simulink model "sm_stewart_platform"  (R2021b)
settings: Solver=ode45  StartTime=0.0  StopTime=40  MaxStep=0.2  RelTol=1e-3  EnableMultiTasking=on
model workspace (MAT data in the model file):
  g_density = 5
values from neighbouring files (symbols this model uses):
  B = zeros(3, 6)    [sm_stewart_platform_setup.m]
  nom_length = params.lower_leg_length + params.upper_leg_length +      2 * params.flange_length    [sm_stewart_platform_setup.m]
  P = rotation3(-pi/3, [0 0 1]) * P    [sm_stewart_platform_setup.m]
  s = cos(angle / 2)    [sm_stewart_platform_setup.m]
undefined symbols (not defined in the file or in its folder): X, Y, Z
libraries: sm_lib x20, sm_stewart_platform_lib x8, nesl_utility x4
(part 2 of 3)

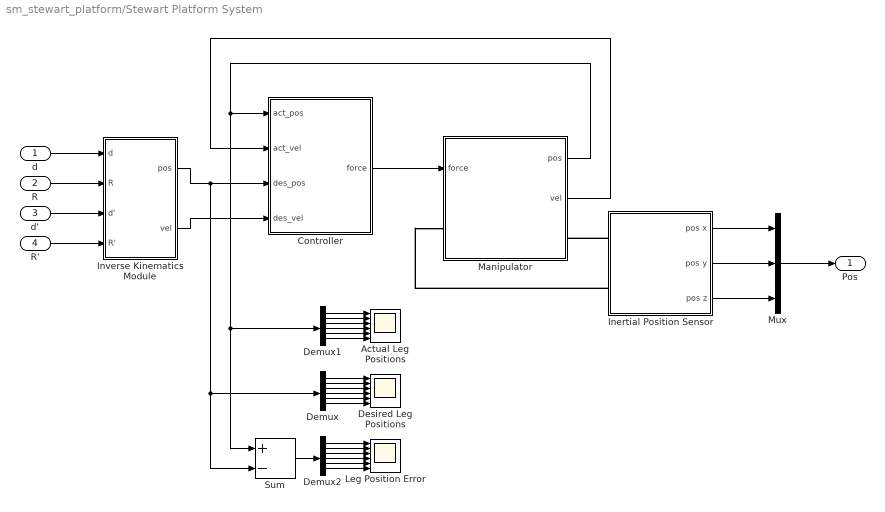
== system sm_stewart_platform/Stewart Platform System ==
  d : Inport
  R : Inport  Port=2
  d' : Inport  Port=3
  R' : Inport  Port=4
  Actual Leg Positions : Scope  NumInputPorts=6
  Controller : Subsystem  mask(PID Controller){Kp=Kp, Ki=Ki, Kd=Kd}
      mask prompts: Kp "Proportional Gain"; Ki "Integral Gain"; Kd "Derivative Gain"
      mask help:
      | Generates an actuation output based on a desired trajectory and an actual trajectory, using a generic proportional-integral-derivative (PID) control law.  The three control gains are specified through parameters.
      |
      | Both the desired and actual trajectories are specified by separate position and velocity input signals.  The controller is generic and can control to trajectories through state spaces of arbitrary dimension; the only requirement is that all four inputs have the same dimension.
      mask Help:
      | A <em>PID Controller</em> generates an actuation output based on a desired trajectory and an actual trajectory, using a generic proportional-integral-derivative (PID) control law.  The three control gains are specified through parameters.
      | 
      | Both the desired and actual trajectories are specified by separate position and velocity input signals.  The controller is generic and can control to trajectories through state spaces of arbitrary dimension; the only requirement is that all four inputs have the same dimension.
      | 
      | This block is not specific to the Stewart platform and could serve in any general purpose control library.  For the Stewart platform application, the trajectories are all through the 6-D leg-position space.
      | 
      | <h3>Gains</h3>
      | 
      | The parameters specify the gains of the controller.
      | 
      | <ul>
      | 
      | <li> <b>Proportional Gain</b> The gain that determines the strength of the control actuation in response to current deviations between actual and desired positions.  This affects the responsiveness of the controller but can lead to instability if set too high.
      | 
      | <li> <b>Integral Gain</b> The gain that determines the strength of the control actuation in response to deviations between actual and desired positions that persist over time.  A nonzero integral term is often necessary to avoid <em>droop</em> (steady-state error).  Higher values reduce the transient response of the controller but can cause overshoot in the controlled position.
      | 
      | <li> <b>Derivative Gain</b> The gain that determines the strength of the control actuation in response to the derivative of the deviations between actual and desired positions.  This is a damping component used to reduce overshoot in the controlled position; the tradeoff is that it reduces the transient response of the controller.  Higher values increase the stiffness of the system and can lead to instability.
      | 
      | </ul>
      | 
      | 
      | <h3>Ports</h3>
      | 
      | <ul>
      | 
      | <li> <b>act_pos</b> The current actual position of the plant.
      | 
      | <li> <b>act_pos</b> The current actual velocity of the plant.  This should be the time derivative of the <em>act_pos</em> signal.
      | 
      | <li> <b>des_pos</b> The current desired position of the plant.
      | 
      | <li> <b>des_pos</b> The current desired velocity of the plant.  This should be the time derivative of the <em>des_pos</em> signal.
      | 
      | </ul>
  Demux : Demux  Outputs=6
  Demux1 : Demux  Outputs=6
  Demux2 : Demux  Outputs=6
  Desired Leg Positions : Scope  NumInputPorts=6
  Inertial Position Sensor : Subsystem
  Inverse Kinematics Module : Subsystem  mask(Stewart Platform Inverse Kinematics){}
      mask help:
      | Performs the essential inverse kinematic computations for a Stewart platform manipulator.
      |
      | Given a desired dynamic state of a Stewart platform manipulator specified by a 3-D rigid transformation from the gripper frame to the base reference frame, and the first time derivative of this transformation, this block computes the positions and velocities of the prismatic primitives of the six cylindrical leg joints necessary to achieve the desired dynamic state.
      mask Help:
      | A <em>Stewart Platform Inverse Kinematics</em> performs the essential inverse kinematic computations for a Stewart platform manipulator.
      | 
      | Given a desired dynamic state of a Stewart platform manipulator specified by a 3-D rigid transformation from the gripper frame to the base reference frame, and the first time derivative of this transformation, this block computes the positions and velocities of the prismatic primitives of the six cylindrical leg joints necessary to achieve the desired dynamic state.
      | 
      | <h3>Manipulator Transformation</h3>
      | 
      | The desired dynamic state of a Stewart platform manipulator may be specified by a single 3-D rigid transformation, called the <em>manipulator transformation</em>, and its time derivative.  The transformation is from <em>gripper</em> frame to <em>base</em> frame coordinates.  The base frame is attached to the base plate of the manipulator.  Its origin is located at the center of the base, and the z-axis points directly upward.  The gripper frame is located somewhere directly above the center of platform plate of the manipulator, and is aligned with the base frame when the positions of the prismatic primitives of all six cylindrical leg joints are equal.
      | 
      | In the following discussions, let <b>R</b> and <b>d</b> specify the rotation matrix and displacement vector, respectively, of the manipulator transformation. That is, <b>d</b> is the origin of the gripper frame specified in base frame coordinates, and the columns of <b>R</b> are the canonical <b>i</b>, <b>j</b>, and <b>k</b> vectors of the gripper frame resolved in base frame coordinates.
      | Let <b>R'</b> and <b>d'</b> be the first time derivatives of <b>R</b> and <b>d</b>, respectively.
      | 
      | <h3>Inverse Kinematics</h3>
      | 
      | Each of the six legs of the manipulator is attached between a pair of universal joints: one on the base plate and one on the platform plate.  Each leg has an internal knee joint with a sensed and actuated prismatic primitive.
      | Let <em>q_i</em> and <em>q_i'</em> be the position and velocity of this primitive on Leg <em>i</em>.  Let <em>L0</em> denote the <em>nominal</em> lengths of the legs.  This is the length of a leg when its prismatic primitive is at the zero position.
      | 
      | The goal of the inverse kinematics computation is to determine the values of <em>q_i</em> and <em>q_i'</em> for i = 1, ..., 6 needed to achieve a particular manipulator transformation and its derivative.
      | 
      | The key to understanding the inverse kinematics computations is to consider the positions of the centers of the pairs of universal joints.  (These points are the centers of the crosspieces visible in the visualization of the manipulator.)
      | 
      | Let <b>b</b>_i and <b>p</b>_i be the 3-D points specifying the center of the universal joints on the base and platform plates, respectively, to which Leg <em>i</em> is connected. <b>b</b>_i is specified in base frame coordinates, and <b>p</b>_i is specified in gripper frame coordinates.  Then the desired position of the prismatic primitive of the knee joint of Leg <em>i</em> is given by
      | 
      | <em>q_i</em> = || <b>R</b> <b>p</b>_i + <b>d</b> - <b>b</b>_i || - <em>L0</em>.
      | 
      | Denote the vector within the norm expression above as <b>o</b>_i (<b>o</b> for <em>offset</em>).
      | 
      | The desired velocity of the prismatic primitive of the knee joint of Leg <em>i</em> is obtained by differentiating the expression for <em>q_i</em>. Noting that <b>p</b>_i, <b>b</b>_i, and <em>L0</em> are constant, the result is:
      | 
      | <em>q_i'</em> = [ (<b>R'</b> <b>p</b>_i + <b>d'</b>) . <b>o</b>_i ] / || <b>o</b>_i ||.
      | 
      | Note that the denominator of this expression is equal to the vector norm in the expression for <em>q_i</em>.
      | 
      | This block computes the values of all six prismatic primitive positions and velocities according to the expressions above.  The computation of the (constant) <b>p</b>_i and <b>b</b>_i points is highly dependent on the manipulator kinematics and done in the mask initialization of the containing <em>Stewart Platform System</em> block.
      | 
      | <h3>Ports</h3>
      | 
      | <ul>
      | 
      | <li> <b>d</b> The displacement vector of the desired manipulator transformation (see above) in units of centimeters.
      | 
      | <li> <b>R</b> The rotation matrix of the desired manipulator transformation (see above).
      | 
      | <li> <b>d'</b> The time derivative of the displacement vector of the desired manipulator transformation in units of centimeters/second.
      | 
      | <li> <b>R'</b> The time derivative of the rotation matrix of the desired manipulator transformation.
      | 
      | <li> <b>pos</b> The computed positions of the prismatic primitives of the six leg joints, as a 6 x 1 vector in units of centimeters.
      | 
      | <li> <b>vel</b> The computed velocities of the prismatic primitives of the six leg joints, as a 6 x 1 vector in units of centimeters/second.
      | 
      | 
      | </ul>
      | 
      | <!--  LocalWords:  ith pos vel
      |  -->
  Leg Position Error : Scope  NumInputPorts=6
  Manipulator : Subsystem  mask(Stewart Platform Manipulator){}
      mask help: Models the mechanical portion of a complete Stewart platform manipulator system: the manipulator itself. Almost all of the Simscape Multibody blocks of the full system are contained in the manipulator subsystem.
      mask Help:
      | A <em>Stewart Platform Manipulator</em> models the mechanical portion of a complete Stewart platform manipulator system: the manipulator itself.  Almost all of the Simscape Multibody blocks of the full system are contained in the manipulator subsystem.
      | 
      | The manipulator subsystem exposes two frames: the world frame, to which the base is anchored, and the gripper frame, which is the frame at the distil end of the end effector.  Typically, a user wants to control the manipulator transformation, which is the 3-D rigid transformation from the gripper frame to the world frame.
      | 
      | The manipulator subsystem has no internal control.  However, it reports the positions and velocities of the prismatic primitives of all six cylindrical leg joints as output signals and takes the actuation forces to be applied to these primitives as input signals.  When connected to an appropriate controller, these signals are sufficient to provide any of a variety of control schemes for the manipulator.
      | 
      | <h3>Parameterization</h3>
      | 
      | The manipulator is highly parameterized.  Most of the physical dimensions of its component pieces can be controlled via parameters.  These parameters are all defined in the containing <em>Stewart Platform System</em>.  The manipulator's parameters are inherited from that block; they are not defined explicitly in this block's mask.  The parameters are also needed for the <em>Stewart Platform Inverse Kinematics</em> block.
      | 
      | See the documentation of the <em>Stewart Platform System</em> block for details.
      | 
      | <h3>Ports</h3>
      | 
      | <ul>
      | 
      | <li> <b>gripper</b> The gripper frame.  This frame is fixed at the distil end of the end effector attached to the platform plate of the Stewart platform manipulator.  It is identified with a frame glyph in the visualization of the manipulator.  Typically, a user of the manipulator wants to control the pose of this frame, with respect to a reference frame such as world.
      | 
      | <li> <b>world</b> The world frame.  This is also the reference frame of the base plate of the Stewart platform manipulator, which is rigidly attached to the world frame.
      | 
      | <li><b>pos</b> The positions of the prismatic primitives of the six leg joints as a 6 x 1 output signal in units of centimeters.
      | 
      | <li><b>vel</b> The velocities of the prismatic primitives of the six leg joints as a 6 x 1 output signal in units of centimeters/second.
      | 
      | <li><b>force</b> The actuation forces applied to the prismatic primitives of the six leg joints as a 6 x 1 input signal in units of Newtons.
      | 
      | </ul>
      | 
      | <!--  LocalWords:  Eff IC Ctrl pos vel
      |  -->
      mask Display:
      | image('sm_stewart_platform_manipulator.png')
      | color('white')
      | port_label('LConn', 1, 'world')
      | port_label('RConn', 1, 'gripper')
      | color('yellow')
      | port_label('Input', 1, 'force')
      | port_label('Output', 1, 'pos')
      | port_label('Output', 2, 'vel')
  Mux : Mux  Inputs=3
  Sum : Sum  Inputs=+-
  Pos : Outport  VectorParamsAs1DForOutWhenUnconnected=off
  wires:
  Manipulator/2(vel) -> Controller/2(act_vel)
  d/1 -> Inverse Kinematics Module/1(d)
  R/1 -> Inverse Kinematics Module/2(R)
  Demux/1 -> Desired Leg Positions/1
  Demux/2 -> Desired Leg Positions/2
  Demux/3 -> Desired Leg Positions/3
  Demux/4 -> Desired Leg Positions/4
  Demux/5 -> Desired Leg Positions/5
  Demux/6 -> Desired Leg Positions/6
  Demux1/1 -> Actual Leg Positions/1
  Demux1/2 -> Actual Leg Positions/2
  Demux1/3 -> Actual Leg Positions/3
  Demux1/4 -> Actual Leg Positions/4
  Demux1/5 -> Actual Leg Positions/5
  Demux1/6 -> Actual Leg Positions/6
  Demux2/1 -> Leg Position Error/1
  Demux2/2 -> Leg Position Error/2
  Demux2/3 -> Leg Position Error/3
  Demux2/4 -> Leg Position Error/4
  Demux2/5 -> Leg Position Error/5
  Demux2/6 -> Leg Position Error/6
  Sum/1 -> Demux2/1
  d'/1 -> Inverse Kinematics Module/3(d')
  R'/1 -> Inverse Kinematics Module/4(R')
  Controller/1(force) -> Manipulator/1(force)
  Manipulator/1(pos) -> Controller/1(act_pos), Demux1/1, Sum/1
  Inertial Position Sensor/1(pos x) -> Mux/1
  Inertial Position Sensor/2(pos y) -> Mux/2
  Inertial Position Sensor/3(pos z) -> Mux/3
  Mux/1 -> Pos/1
  Inverse Kinematics Module/2(vel) -> Controller/4(des_vel)
  Inverse Kinematics Module/1(pos) -> Controller/3(des_pos), Sum/2, Demux/1
  connections:
  Inertial Position Sensor/LConn1 -- Manipulator/RConn1
  Inertial Position Sensor/LConn2 -- Manipulator/LConn1

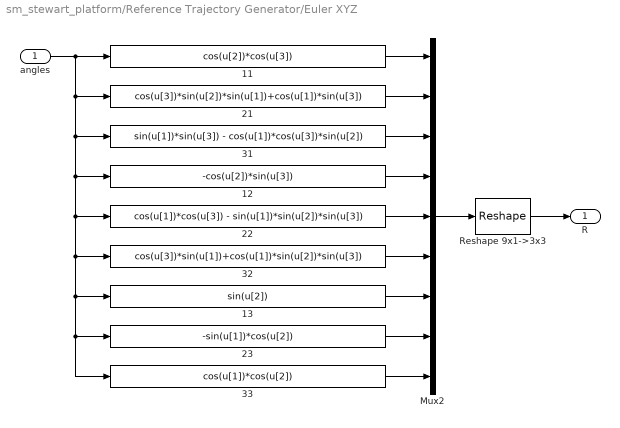
== system sm_stewart_platform/Reference Trajectory Generator/Euler XYZ ==
  angles : Inport
  11 : Fcn  Expr=cos(u[2])*cos(u[3])
  12 : Fcn  Expr=-cos(u[2])*sin(u[3])
  13 : Fcn  Expr=sin(u[2])
  21 : Fcn  Expr=cos(u[3])*sin(u[2])*sin(u[1])+cos(u[1])*sin(u[3])
  22 : Fcn  Expr=cos(u[1])*cos(u[3]) - sin(u[1])*sin(u[2])*sin(u[3])
  23 : Fcn  Expr=-sin(u[1])*cos(u[2])
  31 : Fcn  Expr=sin(u[1])*sin(u[3]) - cos(u[1])*cos(u[3])*sin(u[2])
  32 : Fcn  Expr=cos(u[3])*sin(u[1])+cos(u[1])*sin(u[2])*sin(u[3])
  33 : Fcn  Expr=cos(u[1])*cos(u[2])
  Mux2 : Mux  Inputs=9
  Reshape 9x1->3x3 : Reshape  OutputDimensionality=Customize  OutputDimensions=[3,3]
  R : Outport  VectorParamsAs1DForOutWhenUnconnected=off
  wires:
  angles/1 -> 23/1, 33/1, 13/1, 32/1, 22/1, 12/1, 31/1, 21/1, 11/1
  33/1 -> Mux2/9
  23/1 -> Mux2/8
  13/1 -> Mux2/7
  32/1 -> Mux2/6
  22/1 -> Mux2/5
  12/1 -> Mux2/4
  31/1 -> Mux2/3
  21/1 -> Mux2/2
  11/1 -> Mux2/1
  Mux2/1 -> Reshape 9x1->3x3/1
  Reshape 9x1->3x3/1 -> R/1

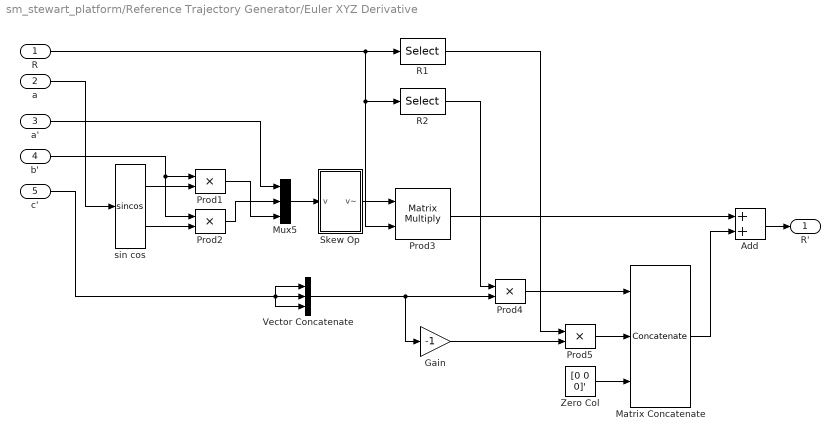
== system sm_stewart_platform/Reference Trajectory Generator/Euler XYZ Derivative ==
  R : Inport
  a : Inport  Port=2
  a' : Inport  Port=3
  b' : Inport  Port=4
  c' : Inport  Port=5
  Add : Sum
  Gain : Gain  Gain=-1
  Matrix Concatenate : Concatenate  NumInputs=3  Mode=Multidimensional array  ConcatenateDimension=2
  Mux5 : Mux  Inputs=3
  Prod{1..2,4..5} (4 alike) : Product  RndMeth=Zero
  Prod3 : Product  Multiplication=Matrix(*)  RndMeth=Zero
  R1 : Selector  NumberOfDimensions=2  InputPortWidth=3  IndexOptions=Select all,Index vector (dialog)  Indices=[1 3],1  OutputSizes=1,1
  R2 : Selector  NumberOfDimensions=2  InputPortWidth=3  IndexOptions=Select all,Index vector (dialog)  Indices=[1 3],2  OutputSizes=1,1
  Skew Op : Subsystem
  Vector Concatenate : Concatenate  NumInputs=3  Mode=Multidimensional array
  Zero Col : Constant  Value=[0 0 0]'
  sin cos : Trigonometry  Operator=sincos
  R' : Outport  VectorParamsAs1DForOutWhenUnconnected=off
  wires:
  a/1 -> sin cos/1
  sin cos/1 -> Prod1/2
  sin cos/2 -> Prod2/2
  b'/1 -> Prod2/1, Prod1/1
  a'/1 -> Mux5/1
  Prod2/1 -> Mux5/2
  Prod1/1 -> Mux5/3
  Mux5/1 -> Skew Op/1(v)
  Vector Concatenate/1 -> Prod4/2, Gain/1
  R2/1 -> Prod4/1
  Gain/1 -> Prod5/2
  Zero Col/1 -> Matrix Concatenate/3
  Prod5/1 -> Matrix Concatenate/2
  Prod4/1 -> Matrix Concatenate/1
  R1/1 -> Prod5/1
  Prod3/1 -> Add/1
  Matrix Concatenate/1 -> Add/2
  Add/1 -> R'/1
  R/1 -> R1/1, Prod3/2, R2/1
  Skew Op/1(v~) -> Prod3/1
  c'/1 -> Vector Concatenate/2, Vector Concatenate/1, Vector Concatenate/3

== system sm_stewart_platform/Reference Trajectory Generator/Rx sinusoid ==
  t : Inport
  Add : Sum  Inputs=|++
  Add2 : Sum  Inputs=++|
  amp1 : Gain  Gain=A
  amp2 : Gain  Gain=w*A*pi/180
  deg2rad : Gain  Gain=pi/180
  freq : Gain  Gain=w
  offset : Constant  Value=k  VectorParams1D=off
  phase : Constant  Value=p  VectorParams1D=off
  sin cos : Trigonometry  Operator=sincos
  f : Outport  VectorParamsAs1DForOutWhenUnconnected=off
  f' : Outport  Port=2  VectorParamsAs1DForOutWhenUnconnected=off
  wires:
  t/1 -> freq/1
  Add/1 -> deg2rad/1
  phase/1 -> Add/2
  amp2/1 -> f'/1
  Add2/1 -> f/1
  offset/1 -> Add2/1
  sin cos/1 -> amp1/1
  sin cos/2 -> amp2/1
  amp1/1 -> Add2/2
  freq/1 -> Add/1
  deg2rad/1 -> sin cos/1

== system sm_stewart_platform/Reference Trajectory Generator/Ry sinusoid ==
  t : Inport
  Add : Sum  Inputs=|++
  Add2 : Sum  Inputs=++|
  amp1 : Gain  Gain=A
  amp2 : Gain  Gain=w*A*pi/180
  deg2rad : Gain  Gain=pi/180
  freq : Gain  Gain=w
  offset : Constant  Value=k  VectorParams1D=off
  phase : Constant  Value=p  VectorParams1D=off
  sin cos : Trigonometry  Operator=sincos
  f : Outport  VectorParamsAs1DForOutWhenUnconnected=off
  f' : Outport  Port=2  VectorParamsAs1DForOutWhenUnconnected=off
  wires:
  t/1 -> freq/1
  Add/1 -> deg2rad/1
  phase/1 -> Add/2
  amp2/1 -> f'/1
  Add2/1 -> f/1
  offset/1 -> Add2/1
  sin cos/1 -> amp1/1
  sin cos/2 -> amp2/1
  amp1/1 -> Add2/2
  freq/1 -> Add/1
  deg2rad/1 -> sin cos/1

== system sm_stewart_platform/Reference Trajectory Generator/Rz sinusoid ==
  t : Inport
  Add : Sum  Inputs=|++
  Add2 : Sum  Inputs=++|
  amp1 : Gain  Gain=A
  amp2 : Gain  Gain=w*A*pi/180
  deg2rad : Gain  Gain=pi/180
  freq : Gain  Gain=w
  offset : Constant  Value=k  VectorParams1D=off
  phase : Constant  Value=p  VectorParams1D=off
  sin cos : Trigonometry  Operator=sincos
  f : Outport  VectorParamsAs1DForOutWhenUnconnected=off
  f' : Outport  Port=2  VectorParamsAs1DForOutWhenUnconnected=off
  wires:
  t/1 -> freq/1
  Add/1 -> deg2rad/1
  phase/1 -> Add/2
  amp2/1 -> f'/1
  Add2/1 -> f/1
  offset/1 -> Add2/1
  sin cos/1 -> amp1/1
  sin cos/2 -> amp2/1
  amp1/1 -> Add2/2
  freq/1 -> Add/1
  deg2rad/1 -> sin cos/1

== system sm_stewart_platform/Reference Trajectory Generator/dx sinusoid ==
  t : Inport
  Add : Sum  Inputs=|++
  Add2 : Sum  Inputs=++|
  amp1 : Gain  Gain=A
  amp2 : Gain  Gain=w*A*pi/180
  deg2rad : Gain  Gain=pi/180
  freq : Gain  Gain=w
  offset : Constant  Value=k  VectorParams1D=off
  phase : Constant  Value=p  VectorParams1D=off
  sin cos : Trigonometry  Operator=sincos
  f : Outport  VectorParamsAs1DForOutWhenUnconnected=off
  f' : Outport  Port=2  VectorParamsAs1DForOutWhenUnconnected=off
  wires:
  t/1 -> freq/1
  Add/1 -> deg2rad/1
  phase/1 -> Add/2
  amp2/1 -> f'/1
  Add2/1 -> f/1
  offset/1 -> Add2/1
  sin cos/1 -> amp1/1
  sin cos/2 -> amp2/1
  amp1/1 -> Add2/2
  freq/1 -> Add/1
  deg2rad/1 -> sin cos/1

== system sm_stewart_platform/Reference Trajectory Generator/dy sinusoid ==
  t : Inport
  Add : Sum  Inputs=|++
  Add2 : Sum  Inputs=++|
  amp1 : Gain  Gain=A
  amp2 : Gain  Gain=w*A*pi/180
  deg2rad : Gain  Gain=pi/180
  freq : Gain  Gain=w
  offset : Constant  Value=k  VectorParams1D=off
  phase : Constant  Value=p  VectorParams1D=off
  sin cos : Trigonometry  Operator=sincos
  f : Outport  VectorParamsAs1DForOutWhenUnconnected=off
  f' : Outport  Port=2  VectorParamsAs1DForOutWhenUnconnected=off
  wires:
  t/1 -> freq/1
  Add/1 -> deg2rad/1
  phase/1 -> Add/2
  amp2/1 -> f'/1
  Add2/1 -> f/1
  offset/1 -> Add2/1
  sin cos/1 -> amp1/1
  sin cos/2 -> amp2/1
  amp1/1 -> Add2/2
  freq/1 -> Add/1
  deg2rad/1 -> sin cos/1

== system sm_stewart_platform/Reference Trajectory Generator/dz sinusoid ==
  t : Inport
  Add : Sum  Inputs=|++
  Add2 : Sum  Inputs=++|
  amp1 : Gain  Gain=A
  amp2 : Gain  Gain=w*A*pi/180
  deg2rad : Gain  Gain=pi/180
  freq : Gain  Gain=w
  offset : Constant  Value=k  VectorParams1D=off
  phase : Constant  Value=p  VectorParams1D=off
  sin cos : Trigonometry  Operator=sincos
  f : Outport  VectorParamsAs1DForOutWhenUnconnected=off
  f' : Outport  Port=2  VectorParamsAs1DForOutWhenUnconnected=off
  wires:
  t/1 -> freq/1
  Add/1 -> deg2rad/1
  phase/1 -> Add/2
  amp2/1 -> f'/1
  Add2/1 -> f/1
  offset/1 -> Add2/1
  sin cos/1 -> amp1/1
  sin cos/2 -> amp2/1
  amp1/1 -> Add2/2
  freq/1 -> Add/1
  deg2rad/1 -> sin cos/1

== system sm_stewart_platform/Stewart Platform System/Controller ==
  act_pos : Inport
  act_vel : Inport  Port=2
  des_pos : Inport  Port=3
  des_vel : Inport  Port=4
  D : Gain  Gain=Kd  SaturateOnIntegerOverflow=on  OutDataTypeStr=Inherit: Same as input  ParamDataTypeStr=Inherit: Same as input
  I : Gain  Gain=Ki  SaturateOnIntegerOverflow=on  OutDataTypeStr=Inherit: Same as input  ParamDataTypeStr=Inherit: Same as input
  Integrator : Integrator  ZeroCross=off
  P : Gain  Gain=Kp  SaturateOnIntegerOverflow=on  OutDataTypeStr=Inherit: Same as input  ParamDataTypeStr=Inherit: Same as input
  Sum : Sum  Inputs=-+|  InputSameDT=on  SaturateOnIntegerOverflow=on  OutDataTypeStr=Inherit: Same as first input
  Sum1 : Sum  Inputs=+++  InputSameDT=on  SaturateOnIntegerOverflow=on  OutDataTypeStr=Inherit: Same as first input
  Sum2 : Sum  Inputs=-+|  InputSameDT=on  SaturateOnIntegerOverflow=on  OutDataTypeStr=Inherit: Same as first input
  force : Outport  VectorParamsAs1DForOutWhenUnconnected=off
  wires:
  Sum2/1 -> D/1
  D/1 -> Sum1/3
  Integrator/1 -> I/1
  P/1 -> Sum1/1
  I/1 -> Sum1/2
  Sum/1 -> P/1, Integrator/1
  act_pos/1 -> Sum/1
  des_pos/1 -> Sum/2
  Sum1/1 -> force/1
  act_vel/1 -> Sum2/1
  des_vel/1 -> Sum2/2

== system sm_stewart_platform/Stewart Platform System/Inertial Position Sensor ==
  note: `
  Pos X Converter : nesl_utility/PS-Simulink Converter  PhysicalDomain=network_engine_domain  SubClassName=ps_output  LeftPortType=input  RightPortType=output  PseudoPeriodic=off  Frequencies=[]  Unit=cm  AffineConversion=off
      settings: SourceProductBaseCode=PW,SS
  Pos Y Converter1 : nesl_utility/PS-Simulink Converter  PhysicalDomain=network_engine_domain  SubClassName=ps_output  LeftPortType=input  RightPortType=output  PseudoPeriodic=off  Frequencies=[]  Unit=cm  AffineConversion=off
      settings: SourceProductBaseCode=PW,SS
  Pos Z Converter2 : nesl_utility/PS-Simulink Converter  PhysicalDomain=network_engine_domain  SubClassName=ps_output  LeftPortType=input  RightPortType=output  PseudoPeriodic=off  Frequencies=[]  Unit=cm  AffineConversion=off
      settings: SourceProductBaseCode=PW,SS
  Transform Sensor : sm_lib/Frames and Transforms/Transform Sensor  MeasurementFrame=World  SenseAngle=off  SenseAxis=off  SenseAngle1=off  SenseAngle2=off  SenseAngle3=off  SenseQ=off  SenseR=off  SenseOmegaX=off  SenseOmegaY=off  SenseOmegaZ=off  SenseOmega1=off  SenseOmega2=off  SenseOmega3=off  SenseQDot=off  SenseRDot=off  SenseAlphaX=off  SenseAlphaY=off  SenseAlphaZ=off  SenseAlpha1=off  SenseAlpha2=off  SenseAlpha3=off  SenseQDDot=off  SenseRDDot=off  SenseX=on  SenseY=on  SenseZ=on  SenseRad=off  SenseAzim=off  SenseDist=off  SenseInc=off  SenseXDot=off  SenseYDot=off  SenseZDot=off  SenseRadDot=off  SenseAzimDot=off  SenseDistDot=off  SenseIncDot=off  SenseXDDot=off  SenseYDDot=off  SenseZDDot=off  SenseRadDDot=off  SenseAzimDDot=off  SenseDistDDot=off  SenseIncDDot=off
  gripper : PMIOPort  Side=Left
  world : PMIOPort  Port=2  Side=Left
  pos x : Outport  VectorParamsAs1DForOutWhenUnconnected=off
  pos y : Outport  Port=2  VectorParamsAs1DForOutWhenUnconnected=off
  pos z : Outport  Port=3  VectorParamsAs1DForOutWhenUnconnected=off
  wires:
  Pos Z Converter2/1 -> pos z/1
  Pos Y Converter1/1 -> pos y/1
  Pos X Converter/1 -> pos x/1
  connections:
  world/RConn1 -- Transform Sensor/LConn1
  gripper/RConn1 -- Transform Sensor/RConn1
  Pos Z Converter2/LConn1 -- Transform Sensor/RConn4
  Pos Y Converter1/LConn1 -- Transform Sensor/RConn3
  Transform Sensor/RConn2 -- Pos X Converter/LConn1

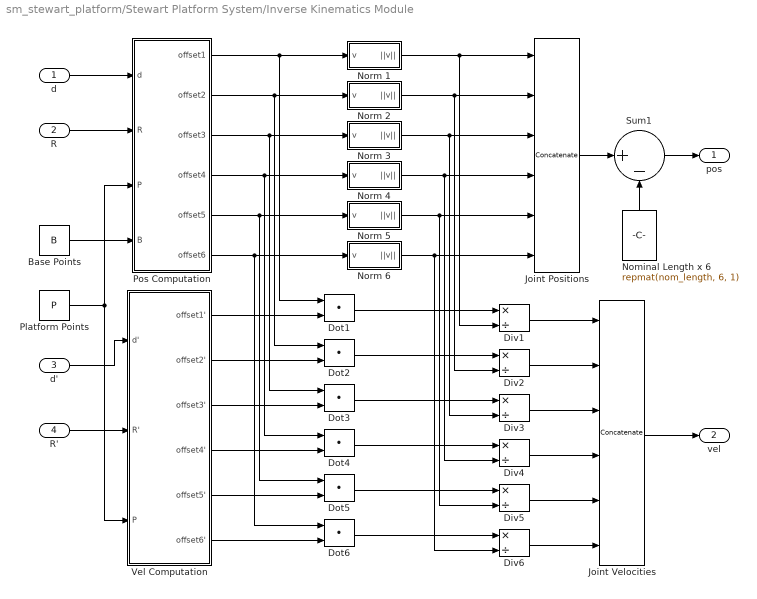
== system sm_stewart_platform/Stewart Platform System/Inverse Kinematics Module ==
  d : Inport
  R : Inport  Port=2
  d' : Inport  Port=3
  R' : Inport  Port=4
  Base Points : Constant  Value=B
  Div{1..6} (6 alike) : Product  Inputs=*/
  Dot{1..6} (6 alike) : DotProduct  OutDataTypeStr=Inherit: Inherit via internal rule
  Joint Positions : Concatenate  NumInputs=6  Mode=Multidimensional array
  Joint Velocities : Concatenate  NumInputs=6  Mode=Multidimensional array
  Nominal Length x 6 : Constant  Value=repmat(nom_length, 6, 1)
  Norm 1 : Subsystem
  Norm 2 : Subsystem
  Norm 3 : Subsystem
  Norm 4 : Subsystem
  Norm 5 : Subsystem
  Norm 6 : Subsystem
  Platform Points : Constant  Value=P
  Pos Computation : Subsystem
  Sum1 : Sum  Inputs=|+-
  Vel Computation : Subsystem
  pos : Outport  VectorParamsAs1DForOutWhenUnconnected=off
  vel : Outport  Port=2  VectorParamsAs1DForOutWhenUnconnected=off
  wires:
  Joint Positions/1 -> Sum1/1
  Nominal Length x 6/1 -> Sum1/2
  Sum1/1 -> pos/1
  d/1 -> Pos Computation/1(d)
  R/1 -> Pos Computation/2(R)
  Base Points/1 -> Pos Computation/4(B)
  Platform Points/1 -> Vel Computation/3(P), Pos Computation/3(P)
  Pos Computation/4(offset4) -> Norm 4/1(v), Dot4/1
  Pos Computation/3(offset3) -> Norm 3/1(v), Dot3/1
  Pos Computation/2(offset2) -> Norm 2/1(v), Dot2/1
  Pos Computation/1(offset1) -> Norm 1/1(v), Dot1/1
  Pos Computation/5(offset5) -> Norm 5/1(v), Dot5/1
  Pos Computation/6(offset6) -> Norm 6/1(v), Dot6/1
  Norm 1/1(||v||) -> Joint Positions/1, Div1/2
  Norm 6/1(||v||) -> Joint Positions/6, Div6/2
  Norm 2/1(||v||) -> Joint Positions/2, Div2/2
  Norm 3/1(||v||) -> Joint Positions/3, Div3/2
  Norm 4/1(||v||) -> Joint Positions/4, Div4/2
  Norm 5/1(||v||) -> Joint Positions/5, Div5/2
  Vel Computation/3(offset3') -> Dot3/2
  Vel Computation/4(offset4') -> Dot4/2
  Vel Computation/2(offset2') -> Dot2/2
  Vel Computation/5(offset5') -> Dot5/2
  Vel Computation/6(offset6') -> Dot6/2
  d'/1 -> Vel Computation/1(d')
  Dot2/1 -> Div2/1
  Dot6/1 -> Div6/1
  Dot5/1 -> Div5/1
  Dot4/1 -> Div4/1
  Dot3/1 -> Div3/1
  Div1/1 -> Joint Velocities/1
  Div2/1 -> Joint Velocities/2
  Div6/1 -> Joint Velocities/6
  Div3/1 -> Joint Velocities/3
  Div4/1 -> Joint Velocities/4
  Div5/1 -> Joint Velocities/5
  Joint Velocities/1 -> vel/1
  R'/1 -> Vel Computation/2(R')
  Vel Computation/1(offset1') -> Dot1/2
  Dot1/1 -> Div1/1

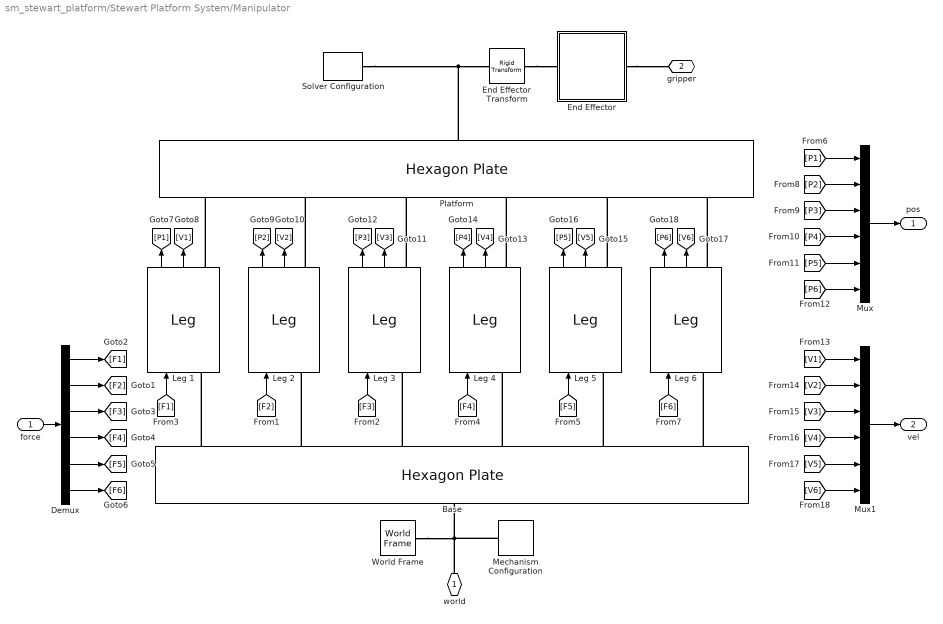
== system sm_stewart_platform/Stewart Platform System/Manipulator ==
  force : Inport
  Base : sm_stewart_platform_lib/Hexagon Plate  kind=base  hex_rad=base_rad  hex_thick=base_thick  hex_skew=hex_skew  flange_sep=2 * leg_rad * cos(pi/6) - flange_thick  flange_len=flange_len  flange_width=flange_width  flange_thick=flange_thick  diffuse=[0.4 0.3 0.2 0.5]  specular=[0 0 0]  shininess=10
      settings: SourceProductBaseCode=MS
  Demux : Demux  Outputs=6
  End Effector : Subsystem  mask(End Effector){grip_height=gripper_height, claw_length=claw_length, claw_width=claw_width, claw_thick=claw_thick, base_thick=end_eff_base_thick}
      mask prompts: grip_height "Gripper Height (cm)"; claw_length "Claw Length (cm)"; claw_width "Claw Width (cm)"; claw_thick "Claw Thickness (cm)"; base_thick "Base Thickness (cm)"
      mask help:
      | Models an end effector attached to the movable platform plate of a Stewart platform manipulator.
      |
      | This end effector comprises a three-claw gripper attached to an approximately triangular base supported by a cylindrical shaft.  The end effector should be rigidly attached to the manipulator platform plate.
      mask Help:
      | An <em>End Effector</em> models an end effector attached to the movable platform
      | plate of a Stewart platform manipulator.
      | 
      | This end effector comprises a three-claw gripper attached to an approximately
      | triangular base supported by a cylindrical shaft.  The end effector should be
      | rigidly attached to the manipulator platform plate at the <em>connection</em>
      | frame.  The <em>gripper</em> frame is centered at the distil end of the gripper
      | jaws.  A coordinate frame glyph marks the pose of the gripper frame in the
      | visualization window.
      | 
      | Stewart platforms are used to manipulate many types of end effectors, tools, and
      | payloads.  This end effector is but one example.
      | 
      | 
      | <h3>Parameters</h3>
      | 
      | <ul>
      | 
      | <li> <b>Gripper Height</b> The vertical distance from the origin of the gripper
      |   frame to the top surface of the movable platform plate of the Stewart platform
      |   manipulator.  This distance must be greater than the base thickness plus the
      |   claw height.  The value determines th e length of the shaft used to support
      |   the gripper.
      | 
      | <li> <b>Claw Length</b> The length (height) of the trapezoidal claws of the
      |   gripper.  This is the distance between the gripper frame and the top surface of
      |   the gripper base.
      | 
      | <li> <b>Claw Width</b> The width of the trapezoidal claws of the gripper where
      |   they attach to the gripper base.  The claws are narrow at their distal ends.
      |   This value is the main factor determining the size of the gripper base; it
      |   also determines the radius of the support shaft.
      | 
      | <li> <b>Claw Thickness</b> The thickness of the trapezoidal claws of the gripper.
      | 
      | <li> <b>Base Thickness</b> The thickness of the triangular gripper base.
      | 
      | </ul>
      | 
      | <h3>Ports</h3>
      | 
      | <ul>
      | 
      | <li> <b>conn</b> The connection frame of the end effector.  This frame is used
      |   to rigidly connect the end effector to the manipulator's moveable platform
      |   plate.  Its origin is at the center of the bottom face of the support shaft,
      |   and its z-axis is aligned with the support shaft axis, pointing up toward the
      |   gripper.  Typically, this frame is attached to a frame at the center of the
      |   top surface of the manipulator platform.
      | 
      | <li> <b>grip</b> The gripper frame of the end effector.  The origin of this
      |   frame is centered between the distil ends of the three gripper claws.  The
      |   z-axis points up, aligned with the gripper's axis of symmetry.  The x- and
      |   y-axes are aligned with the planes of the gripper claws.  The gripper frame
      |   is often the frame that a user of a Stewart platform wants to control.
      | 
      | </ul>
      mask Display:
      | image('sm_stewart_platform_endeffector.png')
      | color('white')
      | port_label('LConn', 1, 'grip')
      | port_label('RConn', 1, 'conn')
  End Effector Transform : sm_lib/Frames and Transforms/Rigid Transform  TranslationMethod=StandardAxis  TranslationStandardOffset=platform_thick / 2  TranslationLengthUnit=cm  TranslationStandardAxis=+Z  TranslationCartesianOffset=[0 0 0]  TranslationROffset=0  TranslationROffsetUnits=m  TranslationZOffset=0  TranslationZOffsetUnits=m  TranslationThetaOffset=0  TranslationThetaOffsetUnits=deg  RotationMethod=StandardAxis  RotationAngleUnits=rad  RotationStandardAxis=+Z  RotationAngle=pi/3  RotationArbitraryAxis=[0 0 1]  FollAlignAxisA=+X  BaseAlignAxisA=+Y  FollAlignAxisB=+Y  BaseAlignAxisB=+Z  RotationSequenceAxes=FollowerAxes  RotationSequence=XYX  RotationSequenceAngles=[0 0 0]  RotationSequenceAnglesUnits=deg  RotationMatrix=[1 0 0; 0 1 0; 0 0 1]
  Leg 1 : sm_stewart_platform_lib/Leg  upper_leg_len=upper_leg_len  lower_leg_len=lower_leg_len  rad=leg_rad  collar_thick=collar_thick  flange_len=flange_len  flange_width=flange_width  flange_thick=flange_thick  asm_offset=lengths(1)
      settings: SourceProductBaseCode=MS
  Leg 2 : sm_stewart_platform_lib/Leg  upper_leg_len=upper_leg_len  lower_leg_len=lower_leg_len  rad=leg_rad  collar_thick=collar_thick  flange_len=flange_len  flange_width=flange_width  flange_thick=flange_thick  asm_offset=lengths(2)
      settings: SourceProductBaseCode=MS
  Leg 3 : sm_stewart_platform_lib/Leg  upper_leg_len=upper_leg_len  lower_leg_len=lower_leg_len  rad=leg_rad  collar_thick=collar_thick  flange_len=flange_len  flange_width=flange_width  flange_thick=flange_thick  asm_offset=lengths(3)
      settings: SourceProductBaseCode=MS
  Leg 4 : sm_stewart_platform_lib/Leg  upper_leg_len=upper_leg_len  lower_leg_len=lower_leg_len  rad=leg_rad  collar_thick=collar_thick  flange_len=flange_len  flange_width=flange_width  flange_thick=flange_thick  asm_offset=lengths(4)
      settings: SourceProductBaseCode=MS
  Leg 5 : sm_stewart_platform_lib/Leg  upper_leg_len=upper_leg_len  lower_leg_len=lower_leg_len  rad=leg_rad  collar_thick=collar_thick  flange_len=flange_len  flange_width=flange_width  flange_thick=flange_thick  asm_offset=lengths(5)
      settings: SourceProductBaseCode=MS
  Leg 6 : sm_stewart_platform_lib/Leg  upper_leg_len=upper_leg_len  lower_leg_len=lower_leg_len  rad=leg_rad  collar_thick=collar_thick  flange_len=flange_len  flange_width=flange_width  flange_thick=flange_thick  asm_offset=lengths(6)
      settings: SourceProductBaseCode=MS
  Mechanism Configuration : sm_lib/Utilities/Mechanism Configuration  UniformGravity=Constant  GravityVector=[0 0 -9.81]  GravityUnits=m/s^2  LinearizationDelta=0.001  JointModeTransitionNonlinearIterations=2
  Mux : Mux  Inputs=6
  Mux1 : Mux  Inputs=6
  Platform : sm_stewart_platform_lib/Hexagon Plate  kind=platform  hex_rad=platform_rad  hex_thick=platform_thick  hex_skew=hex_skew  flange_sep=2 * leg_rad * cos(pi/6) - flange_thick  flange_len=flange_len  flange_width=flange_width  flange_thick=flange_thick  diffuse=[.7 .7 .3 0.75]  specular=[.7 .7 .3 0.75]  shininess=90
      settings: SourceProductBaseCode=MS
  Solver Configuration : nesl_utility/Solver Configuration  PhysicalDomain=network_engine_domain  SubClassName=solver  LeftPortType=input  RightPortType=generic  Tones=[]  Harmonics=[]  SimulateNoise=off  Profile=off  UseLocalSampling=off  EnableSwitchedLinearOptims=on  FrequencyDomain=off  UseCCode=off  RelTol=0.001  AbsTol=1e-06  MinStep=1e-09  ToWorkspace=off  RevertToSquareIcSolve=off  NumHomotopyIterations=100  PhasorMode=off  PhasorModeNumHarmonics=1  DoDC=off  ResidualTolerance=1e-9  UseLocalSolver=off  LocalSolverChoice=NE_BACKWARD_EULER_ADVANCER  LocalSolverSampleTime=.001  DoFixedCost=off  MaxNonlinIter=3  MaxModeIter=2  ComputeImpulses=off  ImpulseIterations=2  LinearAlgebra=Sparse  EquationFormulation=NE_TIME_EF  DelaysMemoryBudget=1024  AutomaticFiltering=on  FilteringTimeConstant=0.001  PartitionStorageMethod=AS_NEEDED  PartitionMemoryBudget=1024  PartitionMethod=FAST
      settings: SourceProductBaseCode=PW,SS
  World Frame : sm_lib/Frames and Transforms/World Frame
  world : PMIOPort  Side=Left
  gripper : PMIOPort  Port=2  Side=Right
  pos : Outport  VectorParamsAs1DForOutWhenUnconnected=off
  vel : Outport  Port=2  VectorParamsAs1DForOutWhenUnconnected=off
  wires:
  Demux/1 -> [F1]
  Demux/2 -> [F2]
  Demux/3 -> [F3]
  Demux/4 -> [F4]
  Demux/5 -> [F5]
  Demux/6 -> [F6]
  [F1] -> Leg 1/1
  [F2] -> Leg 2/1
  [F3] -> Leg 3/1
  [F4] -> Leg 4/1
  [F5] -> Leg 5/1
  [F6] -> Leg 6/1
  force/1 -> Demux/1
  Leg 1/1 -> [P1]
  Leg 1/2 -> [V1]
  Leg 2/1 -> [P2]
  Leg 2/2 -> [V2]
  Leg 3/1 -> [P3]
  Leg 3/2 -> [V3]
  Leg 4/1 -> [P4]
  Leg 4/2 -> [V4]
  Leg 5/1 -> [P5]
  Leg 5/2 -> [V5]
  Leg 6/1 -> [P6]
  Leg 6/2 -> [V6]
  Mux/1 -> pos/1
  [P1] -> Mux/1
  [P2] -> Mux/2
  [P3] -> Mux/3
  [P4] -> Mux/4
  [P5] -> Mux/5
  [P6] -> Mux/6
  [V1] -> Mux1/1
  [V2] -> Mux1/2
  [V3] -> Mux1/3
  [V4] -> Mux1/4
  [V5] -> Mux1/5
  [V6] -> Mux1/6
  Mux1/1 -> vel/1
  connections:
  End Effector/LConn1 -- gripper/RConn1
  Platform/LConn1 -- End Effector Transform/LConn1 -- Solver Configuration/RConn1
  End Effector Transform/RConn1 -- End Effector/RConn1
  Mechanism Configuration/RConn1 -- world/RConn1 -- Base/LConn1 -- World Frame/RConn1
  Base/RConn6 -- Leg 6/LConn1
  Base/RConn5 -- Leg 5/LConn1
  Base/RConn2 -- Leg 2/LConn1
  Base/RConn1 -- Leg 1/LConn1
  Base/RConn3 -- Leg 3/LConn1
  Base/RConn4 -- Leg 4/LConn1
  Leg 1/RConn1 -- Platform/RConn1
  Leg 2/RConn1 -- Platform/RConn2
  Leg 5/RConn1 -- Platform/RConn5
  Leg 6/RConn1 -- Platform/RConn6
  Leg 3/RConn1 -- Platform/RConn3
  Leg 4/RConn1 -- Platform/RConn4

== system sm_stewart_platform/Reference Trajectory Generator/Euler XYZ Derivative/Skew Op ==
  v : Inport
  Demux : Demux  Outputs=3
  Demux1 : Demux  Outputs=3
  Gain : Gain  Gain=-1
  Mux6 : Mux  Inputs=9
  Reshape 9x1->3x3 : Reshape  OutputDimensionality=Customize  OutputDimensions=[3,3]
  Zero : Constant  Value=0
  v~ : Outport  VectorParamsAs1DForOutWhenUnconnected=off
  wires:
  Mux6/1 -> Reshape 9x1->3x3/1
  v/1 -> Demux/1, Gain/1
  Gain/1 -> Demux1/1
  Reshape 9x1->3x3/1 -> v~/1
  Zero/1 -> Mux6/1, Mux6/5, Mux6/9
  Demux/3 -> Mux6/2
  Demux1/2 -> Mux6/3
  Demux1/3 -> Mux6/4
  Demux/1 -> Mux6/6
  Demux/2 -> Mux6/7
  Demux1/1 -> Mux6/8

== system sm_stewart_platform/Stewart Platform System/Inverse Kinematics Module/Norm 1 ==
  v : Inport
  Dot Product : DotProduct  OutDataTypeStr=Inherit: Inherit via internal rule
  Sqrt : Sqrt  SaturateOnIntegerOverflow=on
  ||v|| : Outport  VectorParamsAs1DForOutWhenUnconnected=off
  wires:
  Dot Product/1 -> Sqrt/1
  Sqrt/1 -> ||v||/1
  v/1 -> Dot Product/1, Dot Product/2

== system sm_stewart_platform/Stewart Platform System/Inverse Kinematics Module/Norm 2 ==
  v : Inport
  Dot Product : DotProduct  OutDataTypeStr=Inherit: Inherit via internal rule
  Sqrt : Sqrt  SaturateOnIntegerOverflow=on
  ||v|| : Outport  VectorParamsAs1DForOutWhenUnconnected=off
  wires:
  Dot Product/1 -> Sqrt/1
  Sqrt/1 -> ||v||/1
  v/1 -> Dot Product/1, Dot Product/2

== system sm_stewart_platform/Stewart Platform System/Inverse Kinematics Module/Norm 3 ==
  v : Inport
  Dot Product : DotProduct  OutDataTypeStr=Inherit: Inherit via internal rule
  Sqrt : Sqrt  SaturateOnIntegerOverflow=on
  ||v|| : Outport  VectorParamsAs1DForOutWhenUnconnected=off
  wires:
  Dot Product/1 -> Sqrt/1
  Sqrt/1 -> ||v||/1
  v/1 -> Dot Product/1, Dot Product/2

== system sm_stewart_platform/Stewart Platform System/Inverse Kinematics Module/Norm 4 ==
  v : Inport
  Dot Product : DotProduct  OutDataTypeStr=Inherit: Inherit via internal rule
  Sqrt : Sqrt  SaturateOnIntegerOverflow=on
  ||v|| : Outport  VectorParamsAs1DForOutWhenUnconnected=off
  wires:
  Dot Product/1 -> Sqrt/1
  Sqrt/1 -> ||v||/1
  v/1 -> Dot Product/1, Dot Product/2

== system sm_stewart_platform/Stewart Platform System/Inverse Kinematics Module/Norm 5 ==
  v : Inport
  Dot Product : DotProduct  OutDataTypeStr=Inherit: Inherit via internal rule
  Sqrt : Sqrt  SaturateOnIntegerOverflow=on
  ||v|| : Outport  VectorParamsAs1DForOutWhenUnconnected=off
  wires:
  Dot Product/1 -> Sqrt/1
  Sqrt/1 -> ||v||/1
  v/1 -> Dot Product/1, Dot Product/2

== system sm_stewart_platform/Stewart Platform System/Inverse Kinematics Module/Norm 6 ==
  v : Inport
  Dot Product : DotProduct  OutDataTypeStr=Inherit: Inherit via internal rule
  Sqrt : Sqrt  SaturateOnIntegerOverflow=on
  ||v|| : Outport  VectorParamsAs1DForOutWhenUnconnected=off
  wires:
  Dot Product/1 -> Sqrt/1
  Sqrt/1 -> ||v||/1
  v/1 -> Dot Product/1, Dot Product/2

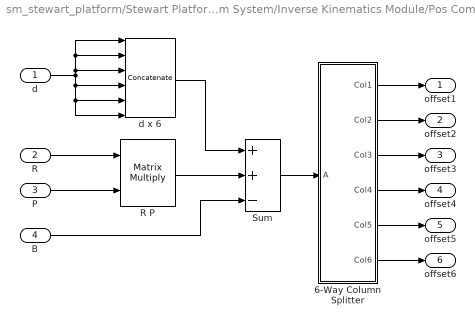
== system sm_stewart_platform/Stewart Platform System/Inverse Kinematics Module/Pos Computation ==
  d : Inport
  R : Inport  Port=2
  P : Inport  Port=3
  B : Inport  Port=4
  6-Way Column Splitter : Subsystem
  R P : Product  Multiplication=Matrix(*)  RndMeth=Zero
  Sum : Sum  Inputs=++-
  d x 6 : Concatenate  NumInputs=6  Mode=Multidimensional array  ConcatenateDimension=2
  offset1 : Outport  VectorParamsAs1DForOutWhenUnconnected=off
  offset2 : Outport  Port=2  VectorParamsAs1DForOutWhenUnconnected=off
  offset3 : Outport  Port=3  VectorParamsAs1DForOutWhenUnconnected=off
  offset4 : Outport  Port=4  VectorParamsAs1DForOutWhenUnconnected=off
  offset5 : Outport  Port=5  VectorParamsAs1DForOutWhenUnconnected=off
  offset6 : Outport  Port=6  VectorParamsAs1DForOutWhenUnconnected=off
  wires:
  d/1 -> d x 6/3, d x 6/2, d x 6/1, d x 6/4, d x 6/5, d x 6/6
  Sum/1 -> 6-Way Column Splitter/1(A)
  P/1 -> R P/2
  6-Way Column Splitter/1(Col1) -> offset1/1
  R/1 -> R P/1
  6-Way Column Splitter/2(Col2) -> offset2/1
  6-Way Column Splitter/3(Col3) -> offset3/1
  6-Way Column Splitter/4(Col4) -> offset4/1
  6-Way Column Splitter/5(Col5) -> offset5/1
  6-Way Column Splitter/6(Col6) -> offset6/1
  d x 6/1 -> Sum/1
  B/1 -> Sum/3
  R P/1 -> Sum/2

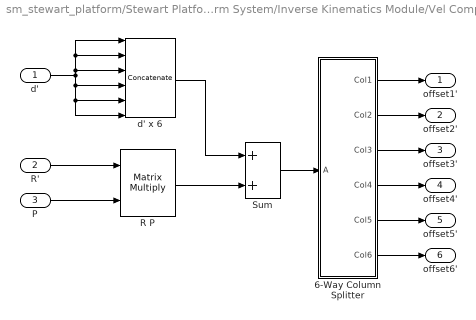
== system sm_stewart_platform/Stewart Platform System/Inverse Kinematics Module/Vel Computation ==
  d' : Inport
  R' : Inport  Port=2
  P : Inport  Port=3
  6-Way Column Splitter : Subsystem
  R P : Product  Multiplication=Matrix(*)  RndMeth=Zero
  Sum : Sum
  d' x 6 : Concatenate  NumInputs=6  Mode=Multidimensional array  ConcatenateDimension=2
  offset1' : Outport  VectorParamsAs1DForOutWhenUnconnected=off
  offset2' : Outport  Port=2  VectorParamsAs1DForOutWhenUnconnected=off
  offset3' : Outport  Port=3  VectorParamsAs1DForOutWhenUnconnected=off
  offset4' : Outport  Port=4  VectorParamsAs1DForOutWhenUnconnected=off
  offset5' : Outport  Port=5  VectorParamsAs1DForOutWhenUnconnected=off
  offset6' : Outport  Port=6  VectorParamsAs1DForOutWhenUnconnected=off
  wires:
  d'/1 -> d' x 6/3, d' x 6/2, d' x 6/1, d' x 6/4, d' x 6/5, d' x 6/6
  Sum/1 -> 6-Way Column Splitter/1(A)
  P/1 -> R P/2
  6-Way Column Splitter/1(Col1) -> offset1'/1
  R'/1 -> R P/1
  6-Way Column Splitter/2(Col2) -> offset2'/1
  6-Way Column Splitter/3(Col3) -> offset3'/1
  6-Way Column Splitter/4(Col4) -> offset4'/1
  6-Way Column Splitter/5(Col5) -> offset5'/1
  6-Way Column Splitter/6(Col6) -> offset6'/1
  d' x 6/1 -> Sum/1
  R P/1 -> Sum/2

== system sm_stewart_platform/Stewart Platform System/Manipulator/End Effector ==
  Gripper : Subsystem  mask(Gripper){claw_length=claw_length, claw_width=claw_width, claw_thick=claw_thick, base_thick=base_thick}
      mask prompts: claw_length "Claw Length (cm)"; claw_width "Claw Width (cm)"; claw_thick "Claw Thickness (cm)"; base_thick "Base Thickness (cm)"
      mask help: Models a three-claw robotic gripper. The gripper is completely rigid and for example purposes only.
      mask init:
      | % Compute cross section vertices of gripper base
      | p3 = [+claw_thick / 2; 2 * claw_width];
      | p4 = [-claw_thick / 2; 2 * claw_width];
      | co = cos(2 * pi / 3);
      | si = sin(2 * pi / 3);
      | R = [co +si; -si co];
      | p1 = R * p3;
      | p2 = R * p4;
      | R = [co -si; +si co];
      | p5 = R * p3;
      | p6 = R * p4;
      mask Help:
      | A <em>Gripper</em> models a three-claw robotic gripper.  The gripper is
      | completely rigid and for demonstration purposes only.
      | 
      | The gripper comprises three claws attached to an approximately triangular base.
      | The gripper exposes two frames: the <em>reference</em> frame at the center of the top
      | surface of the base, and the <em>jaw</em> frame at the center of the distil ends
      | of the claws.
      | 
      | <h3>Parameters</h3>
      | 
      | <ul>
      | 
      | <li> <b>Claw Length</b> The length (height) of the trapezoidal claws of the
      |   gripper.  This is the distance between the gripper frame and the top surface of
      |   the gripper base.
      | 
      | <li> <b>Claw Width</b> The width of the trapezoidal claws of the gripper where
      |   they attach to the gripper base.  The claws are narrower at their distal ends.
      |   This value is the main factor determining the size of the gripper base.
      | 
      | <li> <b>Claw Thickness</b> The thickness of the trapezoidal claws of the gripper.
      | 
      | <li> <b>Base Thickness</b> The thickness of the triangular gripper base.
      | 
      | </ul>
      | 
      | <h3>Ports</h3>
      | 
      | <ul>
      | 
      | <li> <b>ref</b> The reference frame of the gripper.  This frame may be used to
      |   connect the gripper to a robot arm.  Its origin is at the center of the top
      |   face of the triangular base, and its z-axis is aligned with the axis of
      |   symmetry of the gripper, pointing up toward the distil ends of the claws.
      | 
      | <li> <b>jaw</b> The jaw frame of the gripper.  The origin of this frame is
      |   centered between the distil ends of the three gripper claws.  The z-axis
      |   points up, aligned with the gripper's axis of symmetry.  The y-axis lies in
      |   the plane of one of the gripper claws.  This frame is often the frame that
      |   a user of a Stewart platform wants to control.
      | 
      | </ul>
      mask Display:
      | image('sm_stewart_platform_gripper.png')
      | color('white')
      | port_label('LConn', 1, 'ref')
      | port_label('RConn', 1, 'jaw')
  Gripper Transform : sm_lib/Frames and Transforms/Rigid Transform  TranslationMethod=StandardAxis  TranslationStandardOffset=grip_height - claw_length  TranslationLengthUnit=cm  TranslationStandardAxis=+Z  TranslationCartesianOffset=[0 0 0]  TranslationROffset=0  TranslationROffsetUnits=m  TranslationZOffset=0  TranslationZOffsetUnits=m  TranslationThetaOffset=0  TranslationThetaOffsetUnits=deg  RotationMethod=None  RotationAngleUnits=deg  RotationStandardAxis=+Z  RotationAngle=0  RotationArbitraryAxis=[0 0 1]  FollAlignAxisA=+X  BaseAlignAxisA=+Y  FollAlignAxisB=+Y  BaseAlignAxisB=+Z  RotationSequenceAxes=FollowerAxes  RotationSequence=XYX  RotationSequenceAngles=[0 0 0]  RotationSequenceAnglesUnits=deg  RotationMatrix=[1 0 0; 0 1 0; 0 0 1]
  Reference Frame : sm_lib/Frames and Transforms/Reference Frame
  Support Shaft : sm_lib/Body Elements/Cylindrical Solid  GraphicAmbientColor=[.1 .1 .1]  BasedOnType=Density  CenterOfMass=[0 0 0]  CenterOfMassUnits=m  GraphicDiffuseColor=[.5 .5 .6]  CylinderLength=grip_height - (claw_length + claw_thick)  CylinderLengthUnits=cm  CylinderRadius=claw_width / 2  CylinderRadiusUnits=cm  Density=g_density  DensityUnits=g/cm^3  DoExposeReferenceFrame=on  GraphicEmissiveColor=[0.0 0.0 0.0]  ExportEntireGeometry=off  SerializedFrames=<Frames/>  MarkerShape=Sphere  MarkerSize=1  GraphicType=FromGeometry  InertiaType=CalculateFromGeometry  Mass=1  MassUnits=kg  MomentsOfInertia=[1 1 1]  MomentsOfInertiaUnits=kg*m^2  GraphicOpacity=1  ProductsOfInertia=[0 0 0]  ProductsOfInertiaUnits=kg*m^2  GraphicShininess=100  GraphicSpecularColor=[.8 .8 1]  GraphicVisPropType=AdvancedVisualProperties
  Support Transform : sm_lib/Frames and Transforms/Rigid Transform  TranslationMethod=StandardAxis  TranslationStandardOffset=(grip_height - (claw_length + claw_thick)) / 2  TranslationLengthUnit=cm  TranslationStandardAxis=+Z  TranslationCartesianOffset=[0 0 0]  TranslationROffset=0  TranslationROffsetUnits=m  TranslationZOffset=0  TranslationZOffsetUnits=m  TranslationThetaOffset=0  TranslationThetaOffsetUnits=deg  RotationMethod=None  RotationAngleUnits=deg  RotationStandardAxis=+Z  RotationAngle=0  RotationArbitraryAxis=[0 0 1]  FollAlignAxisA=+X  BaseAlignAxisA=+Y  FollAlignAxisB=+Y  BaseAlignAxisB=+Z  RotationSequenceAxes=FollowerAxes  RotationSequence=XYX  RotationSequenceAngles=[0 0 0]  RotationSequenceAnglesUnits=deg  RotationMatrix=[1 0 0; 0 1 0; 0 0 1]
  conn : PMIOPort  Side=Right
  grip : PMIOPort  Port=2  Side=Left
  connections:
  Gripper Transform/LConn1 -- Support Transform/LConn1 -- Reference Frame/RConn1 -- conn/RConn1
  Support Shaft/RConn1 -- Support Transform/RConn1
  Gripper/LConn1 -- Gripper Transform/RConn1
  Gripper/RConn1 -- grip/RConn1
